simulink model "ScriptDemo"  (R2022b)
settings: configuration reference "TmVcThermal_Configuration_sub" (kept outside this file)
undefined symbols (not defined in the file or in its folder): aaaa, bbbb, cTmComprCtrl_D_u8HvacFlowTable_db, cTmComprCtrl_D_u8HvacFlowTable_sw, cTmComprCtrl_n_i16ChillCmpIMax, cTmComprCtrl_n_i16ChillCmpIMin, cTmComprCtrl_n_i16ChillCmpIMin666, cTmComprCtrl_n_i16ChillCmpPMax, cTmComprCtrl_n_i16ChillCmpPMin, cTmComprCtrl_n_i16CmpChillCoolRpmKiMax, cTmComprCtrl_n_i16CmpChillCoolRpmKiMin, cTmComprCtrl_n_i16CmpChillCoolRpmKpMax, cTmComprCtrl_n_i16CmpChillCoolRpmKpMin, cTmComprCtrl_n_i16CmpCoolRpmKiMax, cTmComprCtrl_n_i16CmpCoolRpmKiMin, cTmComprCtrl_n_i16CmpCoolRpmKpMax, cTmComprCtrl_n_i16CmpCoolRpmKpMin, cTmComprCtrl_n_i16SM4CmpHeatKiMax, cTmComprCtrl_n_i16SM4CmpHeatKiMin, cTmComprCtrl_n_i16SM4CmpHeatKpMax, cTmComprCtrl_n_i16SM4CmpHeatKpMin, cTmComprCtrl_n_i16SM5CmpHeatKiMax, cTmComprCtrl_n_i16SM5CmpHeatKiMin, cTmComprCtrl_n_i16SM5CmpHeatKpMax, cTmComprCtrl_n_i16SM5CmpHeatKpMin, cTmComprCtrl_n_i16SM6CmpHeatKiMax, cTmComprCtrl_n_i16SM6CmpHeatKiMin, cTmComprCtrl_n_i16SM6CmpHeatKpMax, cTmComprCtrl_n_i16SM6CmpHeatKpMin, cTmComprCtrl_n_u16CmpMaxSpdFanFltLimt, cTmComprCtrl_n_u16CmpMaxSpdLoSidePFltLimt, cTmComprCtrl_n_u16CmpMaxSpdSensorFltLimt, cTmComprCtrl_n_u16CompMinRpm, cTmComprCtrl_n_u16CompRpmIncThres, cTmComprCtrl_t_u16BattCooltFFPeriod, cTmComprCtrl_t_u16BattCooltPIPeriod, cTmComprCtrl_t_u16CmpCoolFFPeriod, cTmComprCtrl_t_u16CmpCoolPIPeriod, cTmComprCtrl_t_u16CoolCmpChillFFPeriod, cTmComprCtrl_t_u16CoolCmpChillPIPeriod, cTmComprCtrl_t_u16SM4CmpHeatFFPeriod, cTmComprCtrl_t_u16SM4CmpHeatPIPeriod, cTmComprCtrl_t_u16SM5CmpHeatFFPeriod, cTmComprCtrl_t_u16SM5CmpHeatPIPeriod, cTmComprCtrl_t_u16SM6CmpHeatFFPeriod, cTmComprCtrl_t_u16SM6CmpHeatPIPeriod, cTmComprCtrl_Te_EvapClearInteg, cTmComprCtrl_Te_i16HpReqTempSaturoffset, cTmComprCtrl_Te_i16SatLpReplaceDiff, cTmComprCtrl_Te_i16SM3BatDiffStartEvapDecOffset, cTmComprCtrl_Te_i16SM3EvapLo, cTmComprCtrl_Te_i16SM3TBatDiffEntEvapDecOffset, cTmComprCtrl_Te_i16SM3TBatDiffEntEvapDecOffsetQuit, cTmComprCtrl_Te_s32ErrCmpChillPIContinueCoolH, cTmComprCtrl_Te_s32ErrCmpChillPIContinueCoolL, cTmComprCtrl_Te_s32ErrCmpPIContinueChillH, cTmComprCtrl_Te_s32ErrCmpPIContinueChillL, cTmComprCtrl_Te_s32ErrCmpPIContinueCoolH, cTmComprCtrl_Te_s32ErrCmpPIContinueCoolL, cTmComprCtrl_Te_s32ErrCmpPIContinueHeatH ... (+398)
libraries: simulink x846, PCMULib x711, simulink_need_slupdate x4
(part 49 of 49)

== system ScriptDemo/Create/createMerge/Before/SM3SM23/SM3_Ki/SM3SM2LikeKi/Osa/Subsystem4 ==
  In1 : Inport  OutDataTypeStr=int16
  Abs : Abs  OutDataTypeStr=uint16  SaturateOnIntegerOverflow=off
  Add6 : Sum  Inputs=+-  OutDataTypeStr=int16
  Compare To Constant : simulink/Logic and Bit Operations/Compare To Constant  relop=>=  const=0  OutDataTypeStr=boolean
  Compare To Constant1 : simulink/Logic and Bit Operations/Compare To Constant  relop=<=  const=10  OutDataTypeStr=boolean
  Constant6 : Constant  Value=0  OutDataTypeStr=uint16
  Constant7 : Constant  Value=10  OutDataTypeStr=uint16
  Logical Operator : Logic  AllPortsSameDT=off  OutDataTypeStr=boolean
  Switch : Switch  Criteria=u2 ~= 0  SaturateOnIntegerOverflow=off  InputSameDT=off
  Out1 : Outport
  wires:
  Add6/1 -> Switch/1
  Logical Operator/1 -> Switch/2
  Constant6/1 -> Switch/3
  Abs/1 -> Add6/2, Compare To Constant/1, Compare To Constant1/1
  Constant7/1 -> Add6/1
  Switch/1 -> Out1/1
  Compare To Constant1/1 -> Logical Operator/2
  Compare To Constant/1 -> Logical Operator/1
  In1/1 -> Abs/1

== system ScriptDemo/Create/createMerge/Before/SM3SM23/SM3_Ki/SM3SM2LikeKi/Osa/Subsystem5 ==
  In1 : Inport  OutDataTypeStr=int16
  Abs : Abs  OutDataTypeStr=uint16  SaturateOnIntegerOverflow=off
  Add6 : Sum  Inputs=+-  OutDataTypeStr=int16
  Compare To Constant : simulink/Logic and Bit Operations/Compare To Constant  relop=>=  const=0  OutDataTypeStr=boolean
  Compare To Constant1 : simulink/Logic and Bit Operations/Compare To Constant  relop=<=  const=10  OutDataTypeStr=boolean
  Constant6 : Constant  Value=0  OutDataTypeStr=uint16
  Constant7 : Constant  Value=10  OutDataTypeStr=uint16
  Logical Operator : Logic  AllPortsSameDT=off  OutDataTypeStr=boolean
  Switch : Switch  Criteria=u2 ~= 0  SaturateOnIntegerOverflow=off  InputSameDT=off
  Out1 : Outport
  wires:
  Add6/1 -> Switch/1
  Logical Operator/1 -> Switch/2
  Constant6/1 -> Switch/3
  Abs/1 -> Add6/2, Compare To Constant/1, Compare To Constant1/1
  Constant7/1 -> Add6/1
  Switch/1 -> Out1/1
  Compare To Constant1/1 -> Logical Operator/2
  Compare To Constant/1 -> Logical Operator/1
  In1/1 -> Abs/1

== system ScriptDemo/Create/createMerge/Before/SM3SM23/SM3_Ki/SM3SM2LikeKi/Osa/XCP ==
  md_u8Blw : Inport
  Constant1 : Constant  Value=BlwHeatLevel_db
      settings: AttributesFormatString=%<Value>
  Constant28 : Constant  Value=BlwHeatLevel_sw
      settings: AttributesFormatString=%<Value>
  Switch : Switch  Criteria=u2 ~= 0  SaturateOnIntegerOverflow=off  InputSameDT=off
  Out1 : Outport
  wires:
  md_u8Blw/1 -> Switch/3
  Switch/1 -> Out1/1
  Constant28/1 -> Switch/2
  Constant1/1 -> Switch/1

== system ScriptDemo/Create/createMerge/Before/SM3SM23/SM3_Ki/SM3SM2LikeKi/Rec/Subsystem1 ==
  In1 : Inport  OutDataTypeStr=int16
  Abs : Abs  OutDataTypeStr=single  SaturateOnIntegerOverflow=off
  Add6 : Sum  Inputs=+-  OutDataTypeStr=int16
  Compare To Constant : simulink/Logic and Bit Operations/Compare To Constant  relop=>=  const=0  OutDataTypeStr=boolean
  Compare To Constant1 : simulink/Logic and Bit Operations/Compare To Constant  relop=<=  const=10  OutDataTypeStr=boolean
  Constant6 : Constant  Value=0  OutDataTypeStr=uint16
  Constant7 : Constant  Value=10  OutDataTypeStr=uint16
  Logical Operator : Logic  AllPortsSameDT=off  OutDataTypeStr=boolean
  Switch : Switch  Criteria=u2 ~= 0  SaturateOnIntegerOverflow=off  InputSameDT=off
  Out1 : Outport
  wires:
  Add6/1 -> Switch/1
  Logical Operator/1 -> Switch/2
  Constant6/1 -> Switch/3
  Abs/1 -> Add6/2, Compare To Constant/1, Compare To Constant1/1
  Constant7/1 -> Add6/1
  Switch/1 -> Out1/1
  Compare To Constant1/1 -> Logical Operator/2
  Compare To Constant/1 -> Logical Operator/1
  In1/1 -> Abs/1

== system ScriptDemo/Create/createMerge/Before/SM3SM23/SM3_Ki/SM3SM2LikeKi/Rec/Subsystem2 ==
  In1 : Inport  OutDataTypeStr=int16
  Abs : Abs  OutDataTypeStr=uint16  SaturateOnIntegerOverflow=off
  Add6 : Sum  Inputs=+-  OutDataTypeStr=int16
  Compare To Constant : simulink/Logic and Bit Operations/Compare To Constant  relop=>=  const=0  OutDataTypeStr=boolean
  Compare To Constant1 : simulink/Logic and Bit Operations/Compare To Constant  relop=<=  const=10  OutDataTypeStr=boolean
  Constant6 : Constant  Value=0  OutDataTypeStr=uint16
  Constant7 : Constant  Value=10  OutDataTypeStr=uint16
  Logical Operator : Logic  AllPortsSameDT=off  OutDataTypeStr=boolean
  Switch : Switch  Criteria=u2 ~= 0  SaturateOnIntegerOverflow=off  InputSameDT=off
  Out1 : Outport
  wires:
  Add6/1 -> Switch/1
  Logical Operator/1 -> Switch/2
  Constant6/1 -> Switch/3
  Abs/1 -> Add6/2, Compare To Constant/1, Compare To Constant1/1
  Constant7/1 -> Add6/1
  Switch/1 -> Out1/1
  Compare To Constant1/1 -> Logical Operator/2
  Compare To Constant/1 -> Logical Operator/1
  In1/1 -> Abs/1

== system ScriptDemo/Create/createMerge/Before/SM3SM23/SM3_Ki/SM3SM2LikeKi/Rec/Subsystem3 ==
  In1 : Inport  OutDataTypeStr=int16
  Abs : Abs  OutDataTypeStr=uint16  SaturateOnIntegerOverflow=off
  Add6 : Sum  Inputs=+-  OutDataTypeStr=int16
  Compare To Constant : simulink/Logic and Bit Operations/Compare To Constant  relop=>=  const=0  OutDataTypeStr=boolean
  Compare To Constant1 : simulink/Logic and Bit Operations/Compare To Constant  relop=<=  const=10  OutDataTypeStr=boolean
  Constant6 : Constant  Value=0  OutDataTypeStr=uint16
  Constant7 : Constant  Value=10  OutDataTypeStr=uint16
  Logical Operator : Logic  AllPortsSameDT=off  OutDataTypeStr=boolean
  Switch : Switch  Criteria=u2 ~= 0  SaturateOnIntegerOverflow=off  InputSameDT=off
  Out1 : Outport
  wires:
  Add6/1 -> Switch/1
  Logical Operator/1 -> Switch/2
  Constant6/1 -> Switch/3
  Abs/1 -> Add6/2, Compare To Constant/1, Compare To Constant1/1
  Constant7/1 -> Add6/1
  Switch/1 -> Out1/1
  Compare To Constant1/1 -> Logical Operator/2
  Compare To Constant/1 -> Logical Operator/1
  In1/1 -> Abs/1

== system ScriptDemo/Create/createMerge/Before/SM3SM23/SM3_Ki/SM3SM2LikeKi/Rec/Subsystem4 ==
  In1 : Inport  OutDataTypeStr=int16
  Abs : Abs  OutDataTypeStr=uint16  SaturateOnIntegerOverflow=off
  Add6 : Sum  Inputs=+-  OutDataTypeStr=int16
  Compare To Constant : simulink/Logic and Bit Operations/Compare To Constant  relop=>=  const=0  OutDataTypeStr=boolean
  Compare To Constant1 : simulink/Logic and Bit Operations/Compare To Constant  relop=<=  const=10  OutDataTypeStr=boolean
  Constant6 : Constant  Value=0  OutDataTypeStr=uint16
  Constant7 : Constant  Value=10  OutDataTypeStr=uint16
  Logical Operator : Logic  AllPortsSameDT=off  OutDataTypeStr=boolean
  Switch : Switch  Criteria=u2 ~= 0  SaturateOnIntegerOverflow=off  InputSameDT=off
  Out1 : Outport
  wires:
  Add6/1 -> Switch/1
  Logical Operator/1 -> Switch/2
  Constant6/1 -> Switch/3
  Abs/1 -> Add6/2, Compare To Constant/1, Compare To Constant1/1
  Constant7/1 -> Add6/1
  Switch/1 -> Out1/1
  Compare To Constant1/1 -> Logical Operator/2
  Compare To Constant/1 -> Logical Operator/1
  In1/1 -> Abs/1

== system ScriptDemo/Create/createMerge/Before/SM3SM23/SM3_Ki/SM3SM2LikeKi/Rec/Subsystem5 ==
  In1 : Inport  OutDataTypeStr=int16
  Abs : Abs  OutDataTypeStr=uint16  SaturateOnIntegerOverflow=off
  Add6 : Sum  Inputs=+-  OutDataTypeStr=int16
  Compare To Constant : simulink/Logic and Bit Operations/Compare To Constant  relop=>=  const=0  OutDataTypeStr=boolean
  Compare To Constant1 : simulink/Logic and Bit Operations/Compare To Constant  relop=<=  const=10  OutDataTypeStr=boolean
  Constant6 : Constant  Value=0  OutDataTypeStr=uint16
  Constant7 : Constant  Value=10  OutDataTypeStr=uint16
  Logical Operator : Logic  AllPortsSameDT=off  OutDataTypeStr=boolean
  Switch : Switch  Criteria=u2 ~= 0  SaturateOnIntegerOverflow=off  InputSameDT=off
  Out1 : Outport
  wires:
  Add6/1 -> Switch/1
  Logical Operator/1 -> Switch/2
  Constant6/1 -> Switch/3
  Abs/1 -> Add6/2, Compare To Constant/1, Compare To Constant1/1
  Constant7/1 -> Add6/1
  Switch/1 -> Out1/1
  Compare To Constant1/1 -> Logical Operator/2
  Compare To Constant/1 -> Logical Operator/1
  In1/1 -> Abs/1

== system ScriptDemo/Create/createMerge/Before/SM3SM23/SM3_Ki/SM3SM2LikeKi/Rec/XCP ==
  md_u8Blw : Inport
  Constant1 : Constant  Value=BlwHeatLevel_db
      settings: AttributesFormatString=%<Value>
  Constant28 : Constant  Value=BlwHeatLevel_sw
      settings: AttributesFormatString=%<Value>
  Switch : Switch  Criteria=u2 ~= 0  SaturateOnIntegerOverflow=off  InputSameDT=off
  Out1 : Outport
  wires:
  md_u8Blw/1 -> Switch/3
  Switch/1 -> Out1/1
  Constant28/1 -> Switch/2
  Constant1/1 -> Switch/1

== system ScriptDemo/Create/createMerge/Before/SM3SM23/SM3_Kp/SM2Kp/Osa/Subsystem1 ==
  In1 : Inport  OutDataTypeStr=int16
  Abs : Abs  OutDataTypeStr=single  SaturateOnIntegerOverflow=off
  Add6 : Sum  Inputs=+-  OutDataTypeStr=int16
  Compare To Constant : simulink/Logic and Bit Operations/Compare To Constant  relop=>=  const=0  OutDataTypeStr=boolean
  Compare To Constant1 : simulink/Logic and Bit Operations/Compare To Constant  relop=<=  const=10  OutDataTypeStr=boolean
  Constant6 : Constant  Value=0  OutDataTypeStr=uint16
  Constant7 : Constant  Value=10  OutDataTypeStr=uint16
  Logical Operator : Logic  AllPortsSameDT=off  OutDataTypeStr=boolean
  Switch : Switch  Criteria=u2 ~= 0  SaturateOnIntegerOverflow=off  InputSameDT=off
  Out1 : Outport
  wires:
  Add6/1 -> Switch/1
  Logical Operator/1 -> Switch/2
  Constant6/1 -> Switch/3
  Abs/1 -> Add6/2, Compare To Constant/1, Compare To Constant1/1
  Constant7/1 -> Add6/1
  Switch/1 -> Out1/1
  Compare To Constant1/1 -> Logical Operator/2
  Compare To Constant/1 -> Logical Operator/1
  In1/1 -> Abs/1

== system ScriptDemo/Create/createMerge/Before/SM3SM23/SM3_Kp/SM2Kp/Osa/Subsystem2 ==
  In1 : Inport  OutDataTypeStr=int16
  Abs : Abs  OutDataTypeStr=uint16  SaturateOnIntegerOverflow=off
  Add6 : Sum  Inputs=+-  OutDataTypeStr=int16
  Compare To Constant : simulink/Logic and Bit Operations/Compare To Constant  relop=>=  const=0  OutDataTypeStr=boolean
  Compare To Constant1 : simulink/Logic and Bit Operations/Compare To Constant  relop=<=  const=10  OutDataTypeStr=boolean
  Constant6 : Constant  Value=0  OutDataTypeStr=uint16
  Constant7 : Constant  Value=10  OutDataTypeStr=uint16
  Logical Operator : Logic  AllPortsSameDT=off  OutDataTypeStr=boolean
  Switch : Switch  Criteria=u2 ~= 0  SaturateOnIntegerOverflow=off  InputSameDT=off
  Out1 : Outport
  wires:
  Add6/1 -> Switch/1
  Logical Operator/1 -> Switch/2
  Constant6/1 -> Switch/3
  Abs/1 -> Add6/2, Compare To Constant/1, Compare To Constant1/1
  Constant7/1 -> Add6/1
  Switch/1 -> Out1/1
  Compare To Constant1/1 -> Logical Operator/2
  Compare To Constant/1 -> Logical Operator/1
  In1/1 -> Abs/1

== system ScriptDemo/Create/createMerge/Before/SM3SM23/SM3_Kp/SM2Kp/Osa/Subsystem3 ==
  In1 : Inport  OutDataTypeStr=int16
  Abs : Abs  OutDataTypeStr=uint16  SaturateOnIntegerOverflow=off
  Add6 : Sum  Inputs=+-  OutDataTypeStr=int16
  Compare To Constant : simulink/Logic and Bit Operations/Compare To Constant  relop=>=  const=0  OutDataTypeStr=boolean
  Compare To Constant1 : simulink/Logic and Bit Operations/Compare To Constant  relop=<=  const=10  OutDataTypeStr=boolean
  Constant6 : Constant  Value=0  OutDataTypeStr=uint16
  Constant7 : Constant  Value=10  OutDataTypeStr=uint16
  Logical Operator : Logic  AllPortsSameDT=off  OutDataTypeStr=boolean
  Switch : Switch  Criteria=u2 ~= 0  SaturateOnIntegerOverflow=off  InputSameDT=off
  Out1 : Outport
  wires:
  Add6/1 -> Switch/1
  Logical Operator/1 -> Switch/2
  Constant6/1 -> Switch/3
  Abs/1 -> Add6/2, Compare To Constant/1, Compare To Constant1/1
  Constant7/1 -> Add6/1
  Switch/1 -> Out1/1
  Compare To Constant1/1 -> Logical Operator/2
  Compare To Constant/1 -> Logical Operator/1
  In1/1 -> Abs/1

== system ScriptDemo/Create/createMerge/Before/SM3SM23/SM3_Kp/SM2Kp/Osa/Subsystem4 ==
  In1 : Inport  OutDataTypeStr=int16
  Abs : Abs  OutDataTypeStr=uint16  SaturateOnIntegerOverflow=off
  Add6 : Sum  Inputs=+-  OutDataTypeStr=int16
  Compare To Constant : simulink/Logic and Bit Operations/Compare To Constant  relop=>=  const=0  OutDataTypeStr=boolean
  Compare To Constant1 : simulink/Logic and Bit Operations/Compare To Constant  relop=<=  const=10  OutDataTypeStr=boolean
  Constant6 : Constant  Value=0  OutDataTypeStr=uint16
  Constant7 : Constant  Value=10  OutDataTypeStr=uint16
  Logical Operator : Logic  AllPortsSameDT=off  OutDataTypeStr=boolean
  Switch : Switch  Criteria=u2 ~= 0  SaturateOnIntegerOverflow=off  InputSameDT=off
  Out1 : Outport
  wires:
  Add6/1 -> Switch/1
  Logical Operator/1 -> Switch/2
  Constant6/1 -> Switch/3
  Abs/1 -> Add6/2, Compare To Constant/1, Compare To Constant1/1
  Constant7/1 -> Add6/1
  Switch/1 -> Out1/1
  Compare To Constant1/1 -> Logical Operator/2
  Compare To Constant/1 -> Logical Operator/1
  In1/1 -> Abs/1

== system ScriptDemo/Create/createMerge/Before/SM3SM23/SM3_Kp/SM2Kp/Osa/Subsystem5 ==
  In1 : Inport  OutDataTypeStr=int16
  Abs : Abs  OutDataTypeStr=uint16  SaturateOnIntegerOverflow=off
  Add6 : Sum  Inputs=+-  OutDataTypeStr=int16
  Compare To Constant : simulink/Logic and Bit Operations/Compare To Constant  relop=>=  const=0  OutDataTypeStr=boolean
  Compare To Constant1 : simulink/Logic and Bit Operations/Compare To Constant  relop=<=  const=10  OutDataTypeStr=boolean
  Constant6 : Constant  Value=0  OutDataTypeStr=uint16
  Constant7 : Constant  Value=10  OutDataTypeStr=uint16
  Logical Operator : Logic  AllPortsSameDT=off  OutDataTypeStr=boolean
  Switch : Switch  Criteria=u2 ~= 0  SaturateOnIntegerOverflow=off  InputSameDT=off
  Out1 : Outport
  wires:
  Add6/1 -> Switch/1
  Logical Operator/1 -> Switch/2
  Constant6/1 -> Switch/3
  Abs/1 -> Add6/2, Compare To Constant/1, Compare To Constant1/1
  Constant7/1 -> Add6/1
  Switch/1 -> Out1/1
  Compare To Constant1/1 -> Logical Operator/2
  Compare To Constant/1 -> Logical Operator/1
  In1/1 -> Abs/1

== system ScriptDemo/Create/createMerge/Before/SM3SM23/SM3_Kp/SM2Kp/Osa/XCP ==
  md_u8Blw : Inport
  Constant1 : Constant  Value=BlwHeatLevel_db
      settings: AttributesFormatString=%<Value>
  Constant28 : Constant  Value=BlwHeatLevel_sw
      settings: AttributesFormatString=%<Value>
  Switch : Switch  Criteria=u2 ~= 0  SaturateOnIntegerOverflow=off  InputSameDT=off
  Out1 : Outport
  wires:
  md_u8Blw/1 -> Switch/3
  Switch/1 -> Out1/1
  Constant28/1 -> Switch/2
  Constant1/1 -> Switch/1

== system ScriptDemo/Create/createMerge/Before/SM3SM23/SM3_Kp/SM2Kp/Rec/Subsystem1 ==
  In1 : Inport  OutDataTypeStr=int16
  Abs : Abs  OutDataTypeStr=single  SaturateOnIntegerOverflow=off
  Add6 : Sum  Inputs=+-  OutDataTypeStr=int16
  Compare To Constant : simulink/Logic and Bit Operations/Compare To Constant  relop=>=  const=0  OutDataTypeStr=boolean
  Compare To Constant1 : simulink/Logic and Bit Operations/Compare To Constant  relop=<=  const=10  OutDataTypeStr=boolean
  Constant6 : Constant  Value=0  OutDataTypeStr=uint16
  Constant7 : Constant  Value=10  OutDataTypeStr=uint16
  Logical Operator : Logic  AllPortsSameDT=off  OutDataTypeStr=boolean
  Switch : Switch  Criteria=u2 ~= 0  SaturateOnIntegerOverflow=off  InputSameDT=off
  Out1 : Outport
  wires:
  Add6/1 -> Switch/1
  Logical Operator/1 -> Switch/2
  Constant6/1 -> Switch/3
  Abs/1 -> Add6/2, Compare To Constant/1, Compare To Constant1/1
  Constant7/1 -> Add6/1
  Switch/1 -> Out1/1
  Compare To Constant1/1 -> Logical Operator/2
  Compare To Constant/1 -> Logical Operator/1
  In1/1 -> Abs/1

== system ScriptDemo/Create/createMerge/Before/SM3SM23/SM3_Kp/SM2Kp/Rec/Subsystem2 ==
  In1 : Inport  OutDataTypeStr=int16
  Abs : Abs  OutDataTypeStr=uint16  SaturateOnIntegerOverflow=off
  Add6 : Sum  Inputs=+-  OutDataTypeStr=int16
  Compare To Constant : simulink/Logic and Bit Operations/Compare To Constant  relop=>=  const=0  OutDataTypeStr=boolean
  Compare To Constant1 : simulink/Logic and Bit Operations/Compare To Constant  relop=<=  const=10  OutDataTypeStr=boolean
  Constant6 : Constant  Value=0  OutDataTypeStr=uint16
  Constant7 : Constant  Value=10  OutDataTypeStr=uint16
  Logical Operator : Logic  AllPortsSameDT=off  OutDataTypeStr=boolean
  Switch : Switch  Criteria=u2 ~= 0  SaturateOnIntegerOverflow=off  InputSameDT=off
  Out1 : Outport
  wires:
  Add6/1 -> Switch/1
  Logical Operator/1 -> Switch/2
  Constant6/1 -> Switch/3
  Abs/1 -> Add6/2, Compare To Constant/1, Compare To Constant1/1
  Constant7/1 -> Add6/1
  Switch/1 -> Out1/1
  Compare To Constant1/1 -> Logical Operator/2
  Compare To Constant/1 -> Logical Operator/1
  In1/1 -> Abs/1

== system ScriptDemo/Create/createMerge/Before/SM3SM23/SM3_Kp/SM2Kp/Rec/Subsystem3 ==
  In1 : Inport  OutDataTypeStr=int16
  Abs : Abs  OutDataTypeStr=uint16  SaturateOnIntegerOverflow=off
  Add6 : Sum  Inputs=+-  OutDataTypeStr=int16
  Compare To Constant : simulink/Logic and Bit Operations/Compare To Constant  relop=>=  const=0  OutDataTypeStr=boolean
  Compare To Constant1 : simulink/Logic and Bit Operations/Compare To Constant  relop=<=  const=10  OutDataTypeStr=boolean
  Constant6 : Constant  Value=0  OutDataTypeStr=uint16
  Constant7 : Constant  Value=10  OutDataTypeStr=uint16
  Logical Operator : Logic  AllPortsSameDT=off  OutDataTypeStr=boolean
  Switch : Switch  Criteria=u2 ~= 0  SaturateOnIntegerOverflow=off  InputSameDT=off
  Out1 : Outport
  wires:
  Add6/1 -> Switch/1
  Logical Operator/1 -> Switch/2
  Constant6/1 -> Switch/3
  Abs/1 -> Add6/2, Compare To Constant/1, Compare To Constant1/1
  Constant7/1 -> Add6/1
  Switch/1 -> Out1/1
  Compare To Constant1/1 -> Logical Operator/2
  Compare To Constant/1 -> Logical Operator/1
  In1/1 -> Abs/1

== system ScriptDemo/Create/createMerge/Before/SM3SM23/SM3_Kp/SM2Kp/Rec/Subsystem4 ==
  In1 : Inport  OutDataTypeStr=int16
  Abs : Abs  OutDataTypeStr=uint16  SaturateOnIntegerOverflow=off
  Add6 : Sum  Inputs=+-  OutDataTypeStr=int16
  Compare To Constant : simulink/Logic and Bit Operations/Compare To Constant  relop=>=  const=0  OutDataTypeStr=boolean
  Compare To Constant1 : simulink/Logic and Bit Operations/Compare To Constant  relop=<=  const=10  OutDataTypeStr=boolean
  Constant6 : Constant  Value=0  OutDataTypeStr=uint16
  Constant7 : Constant  Value=10  OutDataTypeStr=uint16
  Logical Operator : Logic  AllPortsSameDT=off  OutDataTypeStr=boolean
  Switch : Switch  Criteria=u2 ~= 0  SaturateOnIntegerOverflow=off  InputSameDT=off
  Out1 : Outport
  wires:
  Add6/1 -> Switch/1
  Logical Operator/1 -> Switch/2
  Constant6/1 -> Switch/3
  Abs/1 -> Add6/2, Compare To Constant/1, Compare To Constant1/1
  Constant7/1 -> Add6/1
  Switch/1 -> Out1/1
  Compare To Constant1/1 -> Logical Operator/2
  Compare To Constant/1 -> Logical Operator/1
  In1/1 -> Abs/1

== system ScriptDemo/Create/createMerge/Before/SM3SM23/SM3_Kp/SM2Kp/Rec/Subsystem5 ==
  In1 : Inport  OutDataTypeStr=int16
  Abs : Abs  OutDataTypeStr=uint16  SaturateOnIntegerOverflow=off
  Add6 : Sum  Inputs=+-  OutDataTypeStr=int16
  Compare To Constant : simulink/Logic and Bit Operations/Compare To Constant  relop=>=  const=0  OutDataTypeStr=boolean
  Compare To Constant1 : simulink/Logic and Bit Operations/Compare To Constant  relop=<=  const=10  OutDataTypeStr=boolean
  Constant6 : Constant  Value=0  OutDataTypeStr=uint16
  Constant7 : Constant  Value=10  OutDataTypeStr=uint16
  Logical Operator : Logic  AllPortsSameDT=off  OutDataTypeStr=boolean
  Switch : Switch  Criteria=u2 ~= 0  SaturateOnIntegerOverflow=off  InputSameDT=off
  Out1 : Outport
  wires:
  Add6/1 -> Switch/1
  Logical Operator/1 -> Switch/2
  Constant6/1 -> Switch/3
  Abs/1 -> Add6/2, Compare To Constant/1, Compare To Constant1/1
  Constant7/1 -> Add6/1
  Switch/1 -> Out1/1
  Compare To Constant1/1 -> Logical Operator/2
  Compare To Constant/1 -> Logical Operator/1
  In1/1 -> Abs/1

== system ScriptDemo/Create/createMerge/Before/SM3SM23/SM3_Kp/SM2Kp/Rec/XCP ==
  md_u8Blw : Inport
  Constant1 : Constant  Value=BlwHeatLevel_db
      settings: AttributesFormatString=%<Value>
  Constant28 : Constant  Value=BlwHeatLevel_sw
      settings: AttributesFormatString=%<Value>
  Switch : Switch  Criteria=u2 ~= 0  SaturateOnIntegerOverflow=off  InputSameDT=off
  Out1 : Outport
  wires:
  md_u8Blw/1 -> Switch/3
  Switch/1 -> Out1/1
  Constant28/1 -> Switch/2
  Constant1/1 -> Switch/1

== system ScriptDemo/Create/createMerge/Before/SM3SM23/SM3_Kp/SM3SM2LikeKp/Osa/Subsystem1 ==
  In1 : Inport  OutDataTypeStr=int16
  Abs : Abs  OutDataTypeStr=single  SaturateOnIntegerOverflow=off
  Add6 : Sum  Inputs=+-  OutDataTypeStr=int16
  Compare To Constant : simulink/Logic and Bit Operations/Compare To Constant  relop=>=  const=0  OutDataTypeStr=boolean
  Compare To Constant1 : simulink/Logic and Bit Operations/Compare To Constant  relop=<=  const=10  OutDataTypeStr=boolean
  Constant6 : Constant  Value=0  OutDataTypeStr=uint16
  Constant7 : Constant  Value=10  OutDataTypeStr=uint16
  Logical Operator : Logic  AllPortsSameDT=off  OutDataTypeStr=boolean
  Switch : Switch  Criteria=u2 ~= 0  SaturateOnIntegerOverflow=off  InputSameDT=off
  Out1 : Outport
  wires:
  Add6/1 -> Switch/1
  Logical Operator/1 -> Switch/2
  Constant6/1 -> Switch/3
  Abs/1 -> Add6/2, Compare To Constant/1, Compare To Constant1/1
  Constant7/1 -> Add6/1
  Switch/1 -> Out1/1
  Compare To Constant1/1 -> Logical Operator/2
  Compare To Constant/1 -> Logical Operator/1
  In1/1 -> Abs/1

== system ScriptDemo/Create/createMerge/Before/SM3SM23/SM3_Kp/SM3SM2LikeKp/Osa/Subsystem2 ==
  In1 : Inport  OutDataTypeStr=int16
  Abs : Abs  OutDataTypeStr=uint16  SaturateOnIntegerOverflow=off
  Add6 : Sum  Inputs=+-  OutDataTypeStr=int16
  Compare To Constant : simulink/Logic and Bit Operations/Compare To Constant  relop=>=  const=0  OutDataTypeStr=boolean
  Compare To Constant1 : simulink/Logic and Bit Operations/Compare To Constant  relop=<=  const=10  OutDataTypeStr=boolean
  Constant6 : Constant  Value=0  OutDataTypeStr=uint16
  Constant7 : Constant  Value=10  OutDataTypeStr=uint16
  Logical Operator : Logic  AllPortsSameDT=off  OutDataTypeStr=boolean
  Switch : Switch  Criteria=u2 ~= 0  SaturateOnIntegerOverflow=off  InputSameDT=off
  Out1 : Outport
  wires:
  Add6/1 -> Switch/1
  Logical Operator/1 -> Switch/2
  Constant6/1 -> Switch/3
  Abs/1 -> Add6/2, Compare To Constant/1, Compare To Constant1/1
  Constant7/1 -> Add6/1
  Switch/1 -> Out1/1
  Compare To Constant1/1 -> Logical Operator/2
  Compare To Constant/1 -> Logical Operator/1
  In1/1 -> Abs/1

== system ScriptDemo/Create/createMerge/Before/SM3SM23/SM3_Kp/SM3SM2LikeKp/Osa/Subsystem3 ==
  In1 : Inport  OutDataTypeStr=int16
  Abs : Abs  OutDataTypeStr=uint16  SaturateOnIntegerOverflow=off
  Add6 : Sum  Inputs=+-  OutDataTypeStr=int16
  Compare To Constant : simulink/Logic and Bit Operations/Compare To Constant  relop=>=  const=0  OutDataTypeStr=boolean
  Compare To Constant1 : simulink/Logic and Bit Operations/Compare To Constant  relop=<=  const=10  OutDataTypeStr=boolean
  Constant6 : Constant  Value=0  OutDataTypeStr=uint16
  Constant7 : Constant  Value=10  OutDataTypeStr=uint16
  Logical Operator : Logic  AllPortsSameDT=off  OutDataTypeStr=boolean
  Switch : Switch  Criteria=u2 ~= 0  SaturateOnIntegerOverflow=off  InputSameDT=off
  Out1 : Outport
  wires:
  Add6/1 -> Switch/1
  Logical Operator/1 -> Switch/2
  Constant6/1 -> Switch/3
  Abs/1 -> Add6/2, Compare To Constant/1, Compare To Constant1/1
  Constant7/1 -> Add6/1
  Switch/1 -> Out1/1
  Compare To Constant1/1 -> Logical Operator/2
  Compare To Constant/1 -> Logical Operator/1
  In1/1 -> Abs/1

== system ScriptDemo/Create/createMerge/Before/SM3SM23/SM3_Kp/SM3SM2LikeKp/Osa/Subsystem4 ==
  In1 : Inport  OutDataTypeStr=int16
  Abs : Abs  OutDataTypeStr=uint16  SaturateOnIntegerOverflow=off
  Add6 : Sum  Inputs=+-  OutDataTypeStr=int16
  Compare To Constant : simulink/Logic and Bit Operations/Compare To Constant  relop=>=  const=0  OutDataTypeStr=boolean
  Compare To Constant1 : simulink/Logic and Bit Operations/Compare To Constant  relop=<=  const=10  OutDataTypeStr=boolean
  Constant6 : Constant  Value=0  OutDataTypeStr=uint16
  Constant7 : Constant  Value=10  OutDataTypeStr=uint16
  Logical Operator : Logic  AllPortsSameDT=off  OutDataTypeStr=boolean
  Switch : Switch  Criteria=u2 ~= 0  SaturateOnIntegerOverflow=off  InputSameDT=off
  Out1 : Outport
  wires:
  Add6/1 -> Switch/1
  Logical Operator/1 -> Switch/2
  Constant6/1 -> Switch/3
  Abs/1 -> Add6/2, Compare To Constant/1, Compare To Constant1/1
  Constant7/1 -> Add6/1
  Switch/1 -> Out1/1
  Compare To Constant1/1 -> Logical Operator/2
  Compare To Constant/1 -> Logical Operator/1
  In1/1 -> Abs/1

== system ScriptDemo/Create/createMerge/Before/SM3SM23/SM3_Kp/SM3SM2LikeKp/Osa/Subsystem5 ==
  In1 : Inport  OutDataTypeStr=int16
  Abs : Abs  OutDataTypeStr=uint16  SaturateOnIntegerOverflow=off
  Add6 : Sum  Inputs=+-  OutDataTypeStr=int16
  Compare To Constant : simulink/Logic and Bit Operations/Compare To Constant  relop=>=  const=0  OutDataTypeStr=boolean
  Compare To Constant1 : simulink/Logic and Bit Operations/Compare To Constant  relop=<=  const=10  OutDataTypeStr=boolean
  Constant6 : Constant  Value=0  OutDataTypeStr=uint16
  Constant7 : Constant  Value=10  OutDataTypeStr=uint16
  Logical Operator : Logic  AllPortsSameDT=off  OutDataTypeStr=boolean
  Switch : Switch  Criteria=u2 ~= 0  SaturateOnIntegerOverflow=off  InputSameDT=off
  Out1 : Outport
  wires:
  Add6/1 -> Switch/1
  Logical Operator/1 -> Switch/2
  Constant6/1 -> Switch/3
  Abs/1 -> Add6/2, Compare To Constant/1, Compare To Constant1/1
  Constant7/1 -> Add6/1
  Switch/1 -> Out1/1
  Compare To Constant1/1 -> Logical Operator/2
  Compare To Constant/1 -> Logical Operator/1
  In1/1 -> Abs/1

== system ScriptDemo/Create/createMerge/Before/SM3SM23/SM3_Kp/SM3SM2LikeKp/Osa/XCP ==
  md_u8Blw : Inport
  Constant1 : Constant  Value=BlwHeatLevel_db
      settings: AttributesFormatString=%<Value>
  Constant28 : Constant  Value=BlwHeatLevel_sw
      settings: AttributesFormatString=%<Value>
  Switch : Switch  Criteria=u2 ~= 0  SaturateOnIntegerOverflow=off  InputSameDT=off
  Out1 : Outport
  wires:
  md_u8Blw/1 -> Switch/3
  Switch/1 -> Out1/1
  Constant28/1 -> Switch/2
  Constant1/1 -> Switch/1

== system ScriptDemo/Create/createMerge/Before/SM3SM23/SM3_Kp/SM3SM2LikeKp/Rec/Subsystem1 ==
  In1 : Inport  OutDataTypeStr=int16
  Abs : Abs  OutDataTypeStr=single  SaturateOnIntegerOverflow=off
  Add6 : Sum  Inputs=+-  OutDataTypeStr=int16
  Compare To Constant : simulink/Logic and Bit Operations/Compare To Constant  relop=>=  const=0  OutDataTypeStr=boolean
  Compare To Constant1 : simulink/Logic and Bit Operations/Compare To Constant  relop=<=  const=10  OutDataTypeStr=boolean
  Constant6 : Constant  Value=0  OutDataTypeStr=uint16
  Constant7 : Constant  Value=10  OutDataTypeStr=uint16
  Logical Operator : Logic  AllPortsSameDT=off  OutDataTypeStr=boolean
  Switch : Switch  Criteria=u2 ~= 0  SaturateOnIntegerOverflow=off  InputSameDT=off
  Out1 : Outport
  wires:
  Add6/1 -> Switch/1
  Logical Operator/1 -> Switch/2
  Constant6/1 -> Switch/3
  Abs/1 -> Add6/2, Compare To Constant/1, Compare To Constant1/1
  Constant7/1 -> Add6/1
  Switch/1 -> Out1/1
  Compare To Constant1/1 -> Logical Operator/2
  Compare To Constant/1 -> Logical Operator/1
  In1/1 -> Abs/1

== system ScriptDemo/Create/createMerge/Before/SM3SM23/SM3_Kp/SM3SM2LikeKp/Rec/Subsystem2 ==
  In1 : Inport  OutDataTypeStr=int16
  Abs : Abs  OutDataTypeStr=uint16  SaturateOnIntegerOverflow=off
  Add6 : Sum  Inputs=+-  OutDataTypeStr=int16
  Compare To Constant : simulink/Logic and Bit Operations/Compare To Constant  relop=>=  const=0  OutDataTypeStr=boolean
  Compare To Constant1 : simulink/Logic and Bit Operations/Compare To Constant  relop=<=  const=10  OutDataTypeStr=boolean
  Constant6 : Constant  Value=0  OutDataTypeStr=uint16
  Constant7 : Constant  Value=10  OutDataTypeStr=uint16
  Logical Operator : Logic  AllPortsSameDT=off  OutDataTypeStr=boolean
  Switch : Switch  Criteria=u2 ~= 0  SaturateOnIntegerOverflow=off  InputSameDT=off
  Out1 : Outport
  wires:
  Add6/1 -> Switch/1
  Logical Operator/1 -> Switch/2
  Constant6/1 -> Switch/3
  Abs/1 -> Add6/2, Compare To Constant/1, Compare To Constant1/1
  Constant7/1 -> Add6/1
  Switch/1 -> Out1/1
  Compare To Constant1/1 -> Logical Operator/2
  Compare To Constant/1 -> Logical Operator/1
  In1/1 -> Abs/1

== system ScriptDemo/Create/createMerge/Before/SM3SM23/SM3_Kp/SM3SM2LikeKp/Rec/Subsystem3 ==
  In1 : Inport  OutDataTypeStr=int16
  Abs : Abs  OutDataTypeStr=uint16  SaturateOnIntegerOverflow=off
  Add6 : Sum  Inputs=+-  OutDataTypeStr=int16
  Compare To Constant : simulink/Logic and Bit Operations/Compare To Constant  relop=>=  const=0  OutDataTypeStr=boolean
  Compare To Constant1 : simulink/Logic and Bit Operations/Compare To Constant  relop=<=  const=10  OutDataTypeStr=boolean
  Constant6 : Constant  Value=0  OutDataTypeStr=uint16
  Constant7 : Constant  Value=10  OutDataTypeStr=uint16
  Logical Operator : Logic  AllPortsSameDT=off  OutDataTypeStr=boolean
  Switch : Switch  Criteria=u2 ~= 0  SaturateOnIntegerOverflow=off  InputSameDT=off
  Out1 : Outport
  wires:
  Add6/1 -> Switch/1
  Logical Operator/1 -> Switch/2
  Constant6/1 -> Switch/3
  Abs/1 -> Add6/2, Compare To Constant/1, Compare To Constant1/1
  Constant7/1 -> Add6/1
  Switch/1 -> Out1/1
  Compare To Constant1/1 -> Logical Operator/2
  Compare To Constant/1 -> Logical Operator/1
  In1/1 -> Abs/1

== system ScriptDemo/Create/createMerge/Before/SM3SM23/SM3_Kp/SM3SM2LikeKp/Rec/Subsystem4 ==
  In1 : Inport  OutDataTypeStr=int16
  Abs : Abs  OutDataTypeStr=uint16  SaturateOnIntegerOverflow=off
  Add6 : Sum  Inputs=+-  OutDataTypeStr=int16
  Compare To Constant : simulink/Logic and Bit Operations/Compare To Constant  relop=>=  const=0  OutDataTypeStr=boolean
  Compare To Constant1 : simulink/Logic and Bit Operations/Compare To Constant  relop=<=  const=10  OutDataTypeStr=boolean
  Constant6 : Constant  Value=0  OutDataTypeStr=uint16
  Constant7 : Constant  Value=10  OutDataTypeStr=uint16
  Logical Operator : Logic  AllPortsSameDT=off  OutDataTypeStr=boolean
  Switch : Switch  Criteria=u2 ~= 0  SaturateOnIntegerOverflow=off  InputSameDT=off
  Out1 : Outport
  wires:
  Add6/1 -> Switch/1
  Logical Operator/1 -> Switch/2
  Constant6/1 -> Switch/3
  Abs/1 -> Add6/2, Compare To Constant/1, Compare To Constant1/1
  Constant7/1 -> Add6/1
  Switch/1 -> Out1/1
  Compare To Constant1/1 -> Logical Operator/2
  Compare To Constant/1 -> Logical Operator/1
  In1/1 -> Abs/1

== system ScriptDemo/Create/createMerge/Before/SM3SM23/SM3_Kp/SM3SM2LikeKp/Rec/Subsystem5 ==
  In1 : Inport  OutDataTypeStr=int16
  Abs : Abs  OutDataTypeStr=uint16  SaturateOnIntegerOverflow=off
  Add6 : Sum  Inputs=+-  OutDataTypeStr=int16
  Compare To Constant : simulink/Logic and Bit Operations/Compare To Constant  relop=>=  const=0  OutDataTypeStr=boolean
  Compare To Constant1 : simulink/Logic and Bit Operations/Compare To Constant  relop=<=  const=10  OutDataTypeStr=boolean
  Constant6 : Constant  Value=0  OutDataTypeStr=uint16
  Constant7 : Constant  Value=10  OutDataTypeStr=uint16
  Logical Operator : Logic  AllPortsSameDT=off  OutDataTypeStr=boolean
  Switch : Switch  Criteria=u2 ~= 0  SaturateOnIntegerOverflow=off  InputSameDT=off
  Out1 : Outport
  wires:
  Add6/1 -> Switch/1
  Logical Operator/1 -> Switch/2
  Constant6/1 -> Switch/3
  Abs/1 -> Add6/2, Compare To Constant/1, Compare To Constant1/1
  Constant7/1 -> Add6/1
  Switch/1 -> Out1/1
  Compare To Constant1/1 -> Logical Operator/2
  Compare To Constant/1 -> Logical Operator/1
  In1/1 -> Abs/1

== system ScriptDemo/Create/createMerge/Before/SM3SM23/SM3_Kp/SM3SM2LikeKp/Rec/XCP ==
  md_u8Blw : Inport
  Constant1 : Constant  Value=BlwHeatLevel_db
      settings: AttributesFormatString=%<Value>
  Constant28 : Constant  Value=BlwHeatLevel_sw
      settings: AttributesFormatString=%<Value>
  Switch : Switch  Criteria=u2 ~= 0  SaturateOnIntegerOverflow=off  InputSameDT=off
  Out1 : Outport
  wires:
  md_u8Blw/1 -> Switch/3
  Switch/1 -> Out1/1
  Constant28/1 -> Switch/2
  Constant1/1 -> Switch/1

== system ScriptDemo/Create/createPorts/createPortsGotoUpdateLoop/After/Level3/Level2/Level1/AllowedPower ==
  note: 压缩机不满足开启条件
  note: 压缩机满足开启条件
  note: 压缩机允许功率
  sTmIn_Pw_s32HvCoolgAllwd : Inport
  xTmComprCtrl_B_CompOnReqCompOn : Inport  Port=2
  Compare To Constant : simulink/Logic and Bit Operations/Compare To Constant  relop=>=  const=6500  OutDataTypeStr=boolean
  Compare To Constant1 : simulink/Logic and Bit Operations/Compare To Constant  relop===  const=6500  OutDataTypeStr=boolean
  Constant2 : Constant  Value=0  OutDataTypeStr=single
  Constant4 : Constant  Value=6500  OutDataTypeStr=single
  Switch1 : Switch  Criteria=u2 ~= 0  SaturateOnIntegerOverflow=off  InputSameDT=off
  Switch3 : Switch  Criteria=u2 ~= 0  Threshold=6500  SaturateOnIntegerOverflow=off  InputSameDT=off
  sTmComprCtrl_Pw_s32ElacCmprMaxState : Outport
  yTmComprCtrl_B_HpcCoolgLimd : Outport  Port=2
  wires:
  sTmIn_Pw_s32HvCoolgAllwd/1 -> Switch3/3, Compare To Constant/1
  Constant2/1 -> Switch1/3
  xTmComprCtrl_B_CompOnReqCompOn/1 -> Switch1/2
  Switch3/1 -> Switch1/1
  Switch1/1 -> Compare To Constant1/1, sTmComprCtrl_Pw_s32ElacCmprMaxState/1
  Constant4/1 -> Switch3/1
  Compare To Constant/1 -> Switch3/2
  Compare To Constant1/1 -> yTmComprCtrl_B_HpcCoolgLimd/1

== system ScriptDemo/Create/createPorts/createPortsGotoUpdateLoop/Before/Level3/Level2/Level1/AllowedPower ==
  note: 压缩机不满足开启条件
  note: 压缩机满足开启条件
  note: 压缩机允许功率
  sTmIn_Pw_s32HvCoolgAllwd : Inport
  xTmComprCtrl_B_CompOnReqCompOn : Inport  Port=2
  Compare To Constant : simulink/Logic and Bit Operations/Compare To Constant  relop=>=  const=6500  OutDataTypeStr=boolean
  Compare To Constant1 : simulink/Logic and Bit Operations/Compare To Constant  relop===  const=6500  OutDataTypeStr=boolean
  Constant2 : Constant  Value=0  OutDataTypeStr=single
  Constant4 : Constant  Value=6500  OutDataTypeStr=single
  Switch1 : Switch  Criteria=u2 ~= 0  SaturateOnIntegerOverflow=off  InputSameDT=off
  Switch3 : Switch  Criteria=u2 ~= 0  Threshold=6500  SaturateOnIntegerOverflow=off  InputSameDT=off
  sTmComprCtrl_Pw_s32ElacCmprMaxState : Outport
  yTmComprCtrl_B_HpcCoolgLimd : Outport  Port=2
  wires:
  sTmIn_Pw_s32HvCoolgAllwd/1 -> Switch3/3, Compare To Constant/1
  Constant2/1 -> Switch1/3
  xTmComprCtrl_B_CompOnReqCompOn/1 -> Switch1/2
  Switch3/1 -> Switch1/1
  Switch1/1 -> Compare To Constant1/1, sTmComprCtrl_Pw_s32ElacCmprMaxState/1
  Constant4/1 -> Switch3/1
  Compare To Constant/1 -> Switch3/2
  Compare To Constant1/1 -> yTmComprCtrl_B_HpcCoolgLimd/1

== system ScriptDemo/Create/createMerge/After/SM3SM23/ID26263_SM3Error/SM3HPErr/isNeedOffset/Timer Running2/Unit Delay Resettable External IC1 ==
  u : Inport  OutDataTypeStr=dataType
  IC : Inport  Port=2  OutDataTypeStr=dataType
  R : Inport  Port=3  OutDataTypeStr=boolean
  Constant : Constant  Value=true  OutDataTypeStr=boolean  SampleTime=-1
  Logical Operator : Logic  Operator=NOT  AllPortsSameDT=off  OutDataTypeStr=boolean
  Logical Operator1 : Logic  AllPortsSameDT=off  OutDataTypeStr=boolean
  Switch : Switch  Criteria=u2 ~= 0  InputSameDT=off
  Switch1 : Switch  Criteria=u2 ~= 0  InputSameDT=off
  Unit Delay : UnitDelay  InitialCondition=false  SampleTime=-1  HasFrameUpgradeWarning=on
      settings: AttributesFormatString=X0=%<X0>
  Unit Delay1 : UnitDelay  SampleTime=-1  HasFrameUpgradeWarning=on
      settings: AttributesFormatString=X0=%<X0>
  y : Outport  OutDataTypeStr=dataType
  wires:
  Logical Operator1/1 -> Switch/2
  Unit Delay/1 -> Logical Operator1/1
  Switch1/1 -> Unit Delay1/1
  IC/1 -> Switch/3, Switch1/3
  u/1 -> Switch1/1
  R/1 -> Logical Operator/1
  Logical Operator/1 -> Logical Operator1/2, Switch1/2
  Constant/1 -> Unit Delay/1
  Unit Delay1/1 -> Switch/1
  Switch/1 -> y/1

== system ScriptDemo/Create/createMerge/Before/SM3SM23/ID26263_SM3Error/SM3HPErr/isNeedOffset/Timer Running2/Unit Delay Resettable External IC1 ==
  u : Inport  OutDataTypeStr=dataType
  IC : Inport  Port=2  OutDataTypeStr=dataType
  R : Inport  Port=3  OutDataTypeStr=boolean
  Constant : Constant  Value=true  OutDataTypeStr=boolean  SampleTime=-1
  Logical Operator : Logic  Operator=NOT  AllPortsSameDT=off  OutDataTypeStr=boolean
  Logical Operator1 : Logic  AllPortsSameDT=off  OutDataTypeStr=boolean
  Switch : Switch  Criteria=u2 ~= 0  InputSameDT=off
  Switch1 : Switch  Criteria=u2 ~= 0  InputSameDT=off
  Unit Delay : UnitDelay  InitialCondition=false  SampleTime=-1  HasFrameUpgradeWarning=on
      settings: AttributesFormatString=X0=%<X0>
  Unit Delay1 : UnitDelay  SampleTime=-1  HasFrameUpgradeWarning=on
      settings: AttributesFormatString=X0=%<X0>
  y : Outport  OutDataTypeStr=dataType
  wires:
  Logical Operator1/1 -> Switch/2
  Unit Delay/1 -> Logical Operator1/1
  Switch1/1 -> Unit Delay1/1
  IC/1 -> Switch/3, Switch1/3
  u/1 -> Switch1/1
  R/1 -> Logical Operator/1
  Logical Operator/1 -> Logical Operator1/2, Switch1/2
  Constant/1 -> Unit Delay/1
  Unit Delay1/1 -> Switch/1
  Switch/1 -> y/1

== matlab function ScriptDemo/Create/createHarness/ID31659_OffCodeState/MATLAB Function1 ==
  data: num input; pos output
function pos = findFirstSetBit(num)
    pos = 0;
    if num ~= 0
        pos = 1;
        mask = uint32(1);
        found = false;  % 添加标志位
        while ~found  % 使用pos作为计数器，因为uint32最多32位
            if bitand(num, mask) ~= 0
                found = true;  % 设置标志位
            else
                mask = bitshift(mask, 1);
                pos = pos + 1;
            end
        end
    end
end

== matlab function ScriptDemo/createHarness/ID31659_OffCodeState/MATLAB Function ==
  data: num input; pos output
function pos = findFirstSetBit(num)
    pos = 0;
    if num ~= 0
        pos = 1;
        mask = uint32(1);
        found = false;  % 添加标志位
        while ~found  % 使用pos作为计数器，因为uint32最多32位
            if bitand(num, mask) ~= 0
                found = true;  % 设置标志位
            else
                mask = bitshift(mask, 1);
                pos = pos + 1;
            end
        end
    end
end

== matlab function ScriptDemo/createHarness/ID31659_OffCodeState/MATLAB Function1 ==
  data: num input; pos output
function pos = findFirstSetBit(num)
    pos = 0;
    if num ~= 0
        pos = 1;
        mask = uint32(1);
        found = false;  % 添加标志位
        while ~found  % 使用pos作为计数器，因为uint32最多32位
            if bitand(num, mask) ~= 0
                found = true;  % 设置标志位
            else
                mask = bitshift(mask, 1);
                pos = pos + 1;
            end
        end
    end
end

== matlab function ScriptDemo/Create/createHarness/ID31659_OffCodeState/MATLAB Function2 ==
  data: num input; pos output
function pos = findFirstSetBit(num)
    if num==0
        pos=0;
    else
        pos = 1;
        mask = uint32(1);
        while mask ~= 0
            if bitand(num, mask) ~= 0
                return;
            end
            mask = bitshift(mask, 1);
            pos = pos + 1;
        end
%         pos = 0; % 如果没有找到设置为 1 的位
    end
    
end

== matlab function ScriptDemo/createHarness/ID31659_OffCodeState/MATLAB Function2 ==
  data: num input; pos output
function pos = findFirstSetBit(num)
    if num==0
        pos=0;
    else
        pos = 1;
        mask = uint32(1);
        while mask ~= 0
            if bitand(num, mask) ~= 0
                return;
            end
            mask = bitshift(mask, 1);
            pos = pos + 1;
        end
%         pos = 0; % 如果没有找到设置为 1 的位
    end
    
end

== matlab function ScriptDemo/Create/createHarness/ID31659_OffCodeState/MATLAB Function ==
  data: num input; pos output
function pos = findFirstSetBit(num)
    pos = 0;
    if num ~= 0
        pos = 1;
        mask = uint32(1);
        found = false;  % 添加标志位
        while ~found  % 使用pos作为计数器，因为uint32最多32位
            if bitand(num, mask) ~= 0
                found = true;  % 设置标志位
            else
                mask = bitshift(mask, 1);
                pos = pos + 1;
            end
        end
    end
end
